simulink model "lqrRegulator"  (R2022a)
settings: Solver=VariableStepAuto  StartTime=0.0  StopTime=15  RelTol=1e-3
undefined symbols (not defined in the file or in its folder): A, B, C, g, K_d, l, m, M, Ts
settings Model: Creator=uzivatel  LastModifiedBy=uzivatel

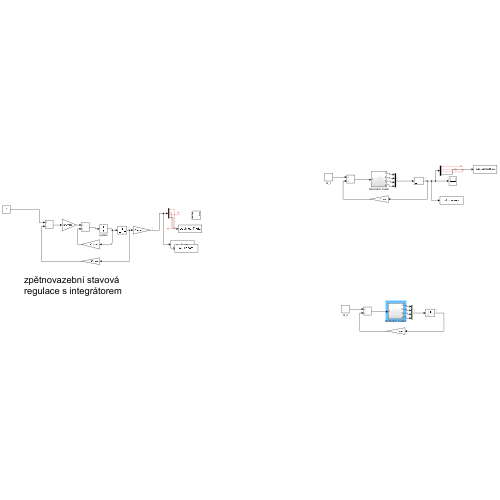
[thumbnail: Simulink's stored preview of the top-level diagram]
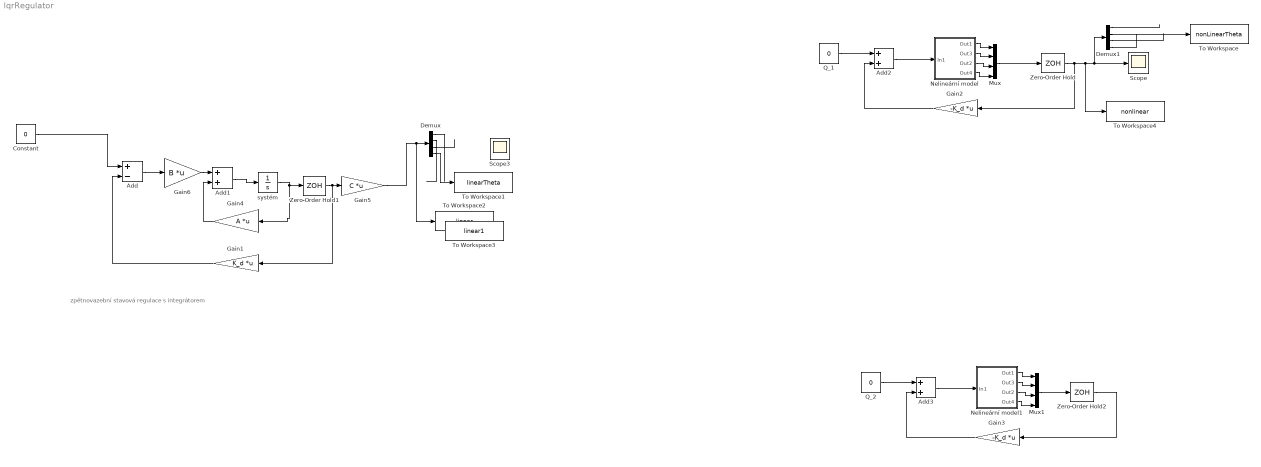
== system lqrRegulator ==
  note: zpětnovazební stavová regulace s integrátorem
  Add : Sum  Inputs=+-
  Add1 : Sum
  Add2 : Sum
  Add3 : Sum
  Constant : Constant  Value=0
  Demux : Demux
  Demux1 : Demux
  Gain1 : Gain  Gain=K_d  Multiplication=Matrix(K*u) (u vector)
  Gain2 : Gain  Gain=-K_d  Multiplication=Matrix(K*u) (u vector)
  Gain3 : Gain  Gain=-K_d  Multiplication=Matrix(K*u) (u vector)
  Gain4 : Gain  Gain=A  Multiplication=Matrix(K*u) (u vector)
  Gain5 : Gain  Gain=C  Multiplication=Matrix(K*u) (u vector)
  Gain6 : Gain  Gain=B  Multiplication=Matrix(K*u) (u vector)
  Mux : Mux
  Mux1 : Mux
  Nelineární model : Subsystem
  Nelineární model1 : Subsystem
  Q_1 : Constant  Value=0
  Q_2 : Constant  Value=0
  Scope : Scope
  Scope3 : Scope  NumInputPorts=2
  To Workspace : ToWorkspace  VariableName=nonLinearTheta  SaveFormat=Timeseries  SampleTime=-1
  To Workspace1 : ToWorkspace  VariableName=linearTheta  SaveFormat=Timeseries  SampleTime=-1
  To Workspace2 : ToWorkspace  VariableName=linear  SaveFormat=Timeseries  SampleTime=-1
  To Workspace3 : ToWorkspace  VariableName=linear1  SaveFormat=Timeseries  SampleTime=-1
  To Workspace4 : ToWorkspace  VariableName=nonlinear  SaveFormat=Timeseries  SampleTime=-1
  Zero-Order Hold : ZeroOrderHold  SampleTime=Ts
  Zero-Order Hold1 : ZeroOrderHold  SampleTime=Ts
  Zero-Order Hold2 : ZeroOrderHold  SampleTime=Ts
  systém : Integrator  InitialCondition=[0;0;pi/6;0]
  wires:
  Gain5/1 -> To Workspace2/1, Demux/1
  Gain1/1 -> Add/2
  Gain4/1 -> Add1/2
  systém/1 -> Zero-Order Hold1/1, Gain4/1
  Gain6/1 -> Add1/1
  Add1/1 -> systém/1
  Add/1 -> Gain6/1
  Constant/1 -> Add/1
  Gain2/1 -> Add2/2
  Nelineární model/1(Out1) -> Mux/1
  Nelineární model/2(Out3) -> Mux/2
  Nelineární model/3(Out2) -> Mux/3
  Nelineární model/4(Out4) -> Mux/4
  Add2/1 -> Nelineární model/1(In1)
  Mux/1 -> Zero-Order Hold/1
  Zero-Order Hold/1 -> Gain2/1, To Workspace4/1, Demux1/1, Scope/1
  Zero-Order Hold1/1 -> Gain1/1, Gain5/1
  Demux1/3 -> ?
  Demux/3 -> ?
  Demux1/1 -> ?
  Demux/1 -> ?
  Demux/2 -> ?
  Demux1/2 -> ?
  Demux/4 -> To Workspace1/1
  Demux1/4 -> To Workspace/1
  Q_1/1 -> Add2/1
  Q_2/1 -> Add3/1
  Nelineární model1/4(Out4) -> Mux1/4
  Zero-Order Hold2/1 -> Gain3/1
  Add3/1 -> Nelineární model1/1(In1)
  Nelineární model1/3(Out2) -> Mux1/3
  Mux1/1 -> Zero-Order Hold2/1
  Nelineární model1/2(Out3) -> Mux1/2
  Nelineární model1/1(Out1) -> Mux1/1
  Gain3/1 -> Add3/2

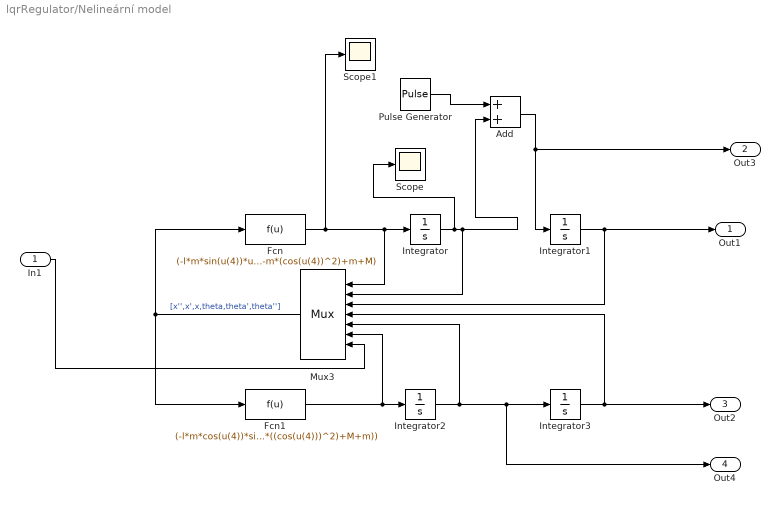
== system lqrRegulator/Nelineární model ==
  In1 : Inport
  Add : Sum
  Fcn : Fcn  Expr=(-l*m*sin(u(4))*u(5)^2+u(7)-m*g*cos(u(4))*sin(u(4)))/(-m*(cos(u(4))^2)+m+M)
  Fcn1 : Fcn  Expr=(-l*m*cos(u(4))*sin(u(4))*u(5)^2+u(7)*cos(u(4))-g*m*sin(u(4))-M*g*sin(u(4)))/(l*(-m*((cos(u(4)))^2)+M+m))
  Integrator : Integrator
  Integrator1 : Integrator
  Integrator2 : Integrator
  Integrator3 : Integrator  InitialCondition=pi/6
  Mux3 : Mux  Inputs=7
      settings: DisplayOption=signals
  Pulse Generator : DiscretePulseGenerator  PulseType=Time based  Amplitude=0  PulseWidth=5
  Scope : Scope
  Scope1 : Scope
  Out1 : Outport
  Out3 : Outport  Port=2
  Out2 : Outport  Port=3
  Out4 : Outport  Port=4
  wires:
  Integrator/1 -> Scope/1, Mux3/2, Add/2
  Fcn1/1 -> Mux3/6, Integrator2/1
  Mux3/1 -> Fcn/1, Fcn1/1  "[x'',x',x,theta,theta',theta'']"
  Integrator1/1 -> Out1/1, Mux3/3
  Integrator3/1 -> Out2/1, Mux3/4
  Integrator2/1 -> Mux3/5, Out4/1, Integrator3/1
  Fcn/1 -> Mux3/1, Integrator/1, Scope1/1
  In1/1 -> Mux3/7
  Pulse Generator/1 -> Add/1
  Add/1 -> Integrator1/1, Out3/1

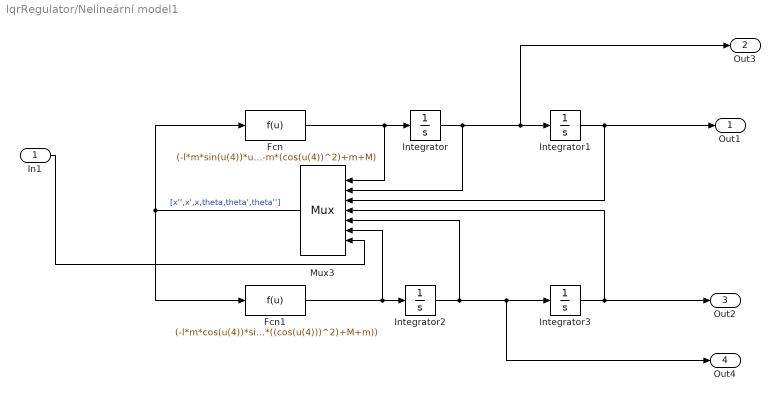
== system lqrRegulator/Nelineární model1 ==
  In1 : Inport
  Fcn : Fcn  Expr=(-l*m*sin(u(4))*u(5)^2+u(7)-m*g*cos(u(4))*sin(u(4)))/(-m*(cos(u(4))^2)+m+M)
  Fcn1 : Fcn  Expr=(-l*m*cos(u(4))*sin(u(4))*u(5)^2+u(7)*cos(u(4))-g*m*sin(u(4))-M*g*sin(u(4)))/(l*(-m*((cos(u(4)))^2)+M+m))
  Integrator : Integrator
  Integrator1 : Integrator
  Integrator2 : Integrator
  Integrator3 : Integrator  InitialCondition=pi/6
  Mux3 : Mux  Inputs=7
      settings: DisplayOption=signals
  Out1 : Outport
  Out3 : Outport  Port=2
  Out2 : Outport  Port=3
  Out4 : Outport  Port=4
  wires:
  Integrator/1 -> Out3/1, Integrator1/1, Mux3/2
  Fcn1/1 -> Mux3/6, Integrator2/1
  Mux3/1 -> Fcn/1, Fcn1/1  "[x'',x',x,theta,theta',theta'']"
  Integrator1/1 -> Out1/1, Mux3/3
  Integrator3/1 -> Out2/1, Mux3/4
  Integrator2/1 -> Mux3/5, Out4/1, Integrator3/1
  Fcn/1 -> Mux3/1, Integrator/1
  In1/1 -> Mux3/7
